simulink model "MMS_ESC_K_B_SM"  (R2019b)
settings: Solver=ode4  StartTime=par.sym.TStart  StopTime=par.sym.TStop  FixedStep=par.sym.max_dt  MaxStep=par.sym.max_dt  RelTol=1e-3
undefined symbols (not defined in the file): b, B_0, beta_B, beta_K, k, K_0, k_B, k_K, m, N_delay, par, rho_B, rho_K, T_tran, W_K, w_wav
libraries: simulink x2
settings Model: Creator=Vitù  LastModifiedBy=User
settings DataIOCC: SaveFormat=Array  SaveOutput=off  SignalLogging=off  DSMLogging=off  ReturnWorkspaceOutputs=off  TimeSaveName=TIME  OutputSaveName=Yout  OutputOption=SpecifiedOutputTimes  OutputTimes=[par.sym.TStart:par.sym.Outputdt:par.sym.TStop]
settings OptimizationCC: ExpressionDepthLimit=2147483647  LifeSpan=inf
settings DebuggingCC: UnderspecifiedInitializationDetection=Classic  MergeDetectMultiDrivingBlocksExec=none  SolverPrmCheckMsg=warning  AllowSymbolicDim=off  StateNameClashWarn=warning  SFUnexpectedBacktrackingDiag=warning  SFNoUnconditionalDefaultTransitionDiag=warning  SFExecutionAtInitializationDiag=none  ArithmeticOperatorsInVariantConditions=warning
settings HardwareCC: ProdBitPerPointer=32  ProdBitPerSizeT=32  ProdBitPerPtrDiffT=32  ProdLargestAtomicFloat=None  ProdIntDivRoundTo=Undefined  ProdEndianess=Unspecified  ProdWordSize=32  ProdHWDeviceType=32-bit Generic
settings ModelReferenceCC: PropagateSignalLabelsOutOfModel=off
settings SFSimCC: SimUseLocalCustomCode=off  CustomCodeUndefinedFunction=UseInterfaceOnly
settings RTWCC: RTWUseLocalCustomCode=off
settings CodeAppCC: StateflowObjectComments=on
settings GRTTargetCC: TargetLangStandard=C89/C90 (ANSI)  GeneratePreprocessorConditionals=Disable all
settings ConfigComp: CovMetricSettings=dw  CovHtmlReporting=on  CovSaveCumulativeToWorkspaceVar=on  CovSaveSingleToWorkspaceVar=on  CovExternalEMLEnable=off  CovSFcnEnable=off
settings SimscapeCC: SimscapeNormalizeSystem=off
settings ConfigurationSet: Description=SimMechanics 2G

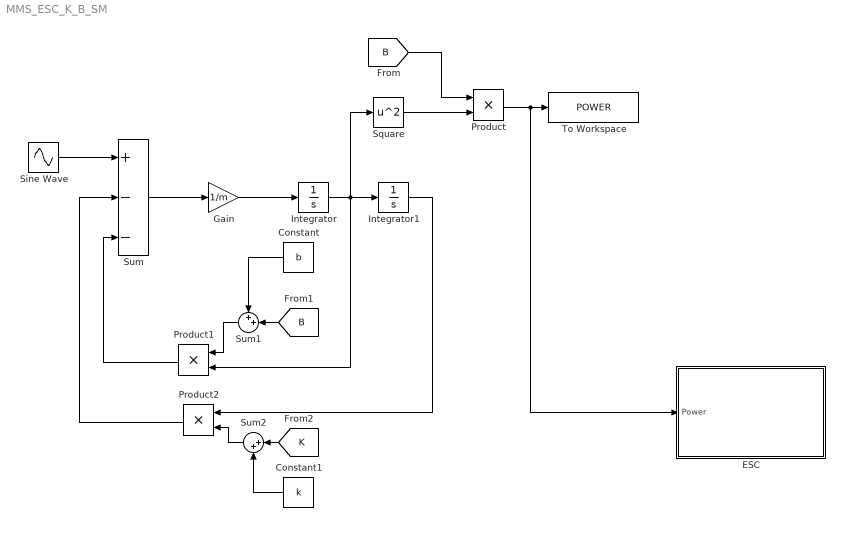
== system MMS_ESC_K_B_SM ==
  Constant : Constant  Value=b
  Constant1 : Constant  Value=k
  ESC : Subsystem
  Gain : Gain  Gain=1/m
  Integrator : Integrator
  Integrator1 : Integrator
  Product : Product
  Product1 : Product
  Product2 : Product
  Sine Wave : Sin  Amplitude=par.H  Frequency=w_wav  SampleTime=0
  Square : Math  Operator=square  SignedPower=off  SaturateOnIntegerOverflow=on
  Sum : Sum  Inputs=+--
  Sum1 : Sum  Inputs=++|
  Sum2 : Sum  Inputs=|++
  To Workspace : ToWorkspace  VariableName=POWER  SampleTime=-1
  wires:
  Integrator1/1 -> Product2/1
  Product/1 -> ESC/1(Power), To Workspace/1
  Product1/1 -> Sum/3
  Gain/1 -> Integrator/1
  Square/1 -> Product/2
  Sum/1 -> Gain/1
  Integrator/1 -> Product1/2, Square/1, Integrator1/1
  Product2/1 -> Sum/2
  Sine Wave/1 -> Sum/1
  [B] -> Product/1
  [B] -> Sum1/2
  Sum1/1 -> Product1/1
  Constant/1 -> Sum1/1
  [K] -> Sum2/1
  Sum2/1 -> Product2/2
  Constant1/1 -> Sum2/2

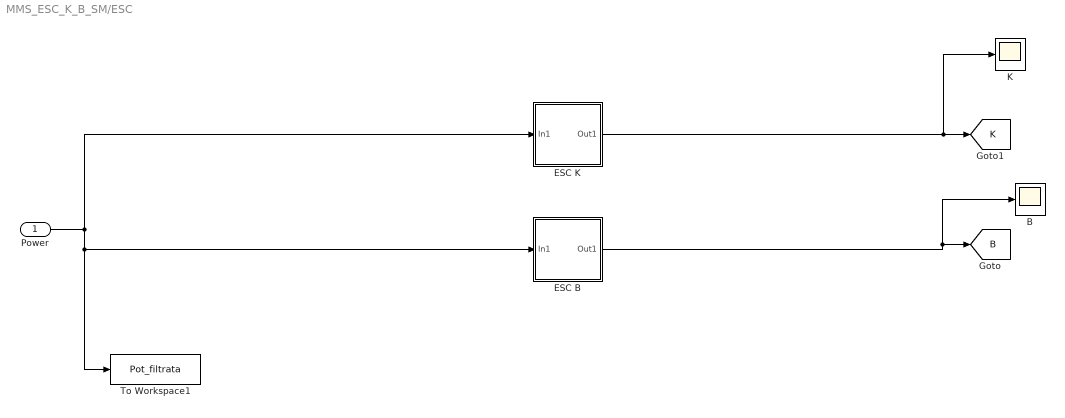
== system MMS_ESC_K_B_SM/ESC ==
  Power : Inport
  B : Scope
  ESC B : Subsystem
  ESC K : Subsystem
  K : Scope
  To Workspace1 : ToWorkspace  VariableName=Pot_filtrata  SampleTime=-1
  tag scope: B=global, K=global
  wires:
  ESC B/1(Out1) -> B/1, [B]
  ESC K/1(Out1) -> K/1, [K]
  Power/1 -> To Workspace1/1, ESC B/1(In1), ESC K/1(In1)

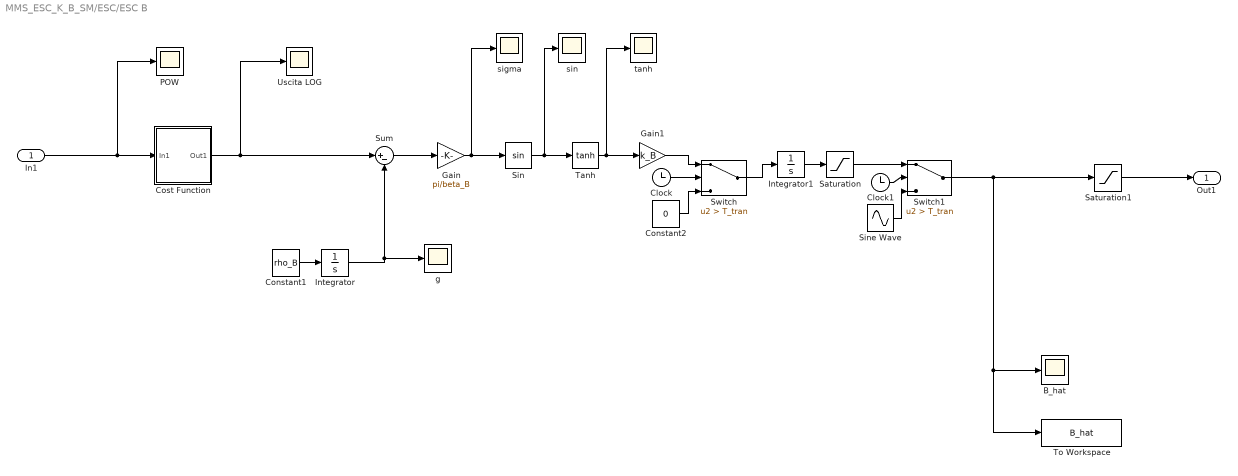
== system MMS_ESC_K_B_SM/ESC/ESC B ==
  In1 : Inport
  B_hat : Scope
  Clock : Clock
  Clock1 : Clock
  Constant1 : Constant  Value=rho_B
  Constant2 : Constant  Value=0
  Cost Function : Subsystem
  Gain : Gain  Gain=pi/beta_B
  Gain1 : Gain  Gain=k_B
  Integrator : Integrator
  Integrator1 : Integrator  InitialCondition=B_0
  POW : Scope
  Saturation : Saturate  UpperLimit=inf  LowerLimit=5
  Saturation1 : Saturate  UpperLimit=inf  LowerLimit=-b
  Sin : Trigonometry
  Sine Wave : Sin  Amplitude=5  Bias=B_0  Frequency=w_wav  SampleTime=0
  Sum : Sum  Inputs=|+-
  Switch : Switch  Criteria=u2 > Threshold  Threshold=T_tran
  Switch1 : Switch  Criteria=u2 > Threshold  Threshold=T_tran
  Tanh : Trigonometry  Operator=tanh
  To Workspace : ToWorkspace  VariableName=B_hat  SampleTime=-1
  Uscita LOG : Scope
  g : Scope
  sigma : Scope
  sin : Scope
  tanh : Scope
  Out1 : Outport
  wires:
  Integrator/1 -> g/1, Sum/2
  Gain/1 -> sigma/1, Sin/1
  Switch1/1 -> Saturation1/1, To Workspace/1, B_hat/1
  Sin/1 -> sin/1, Tanh/1
  Tanh/1 -> tanh/1, Gain1/1
  Switch/1 -> Integrator1/1
  Cost Function/1(Out1) -> Uscita LOG/1, Sum/1
  Sine Wave/1 -> Switch1/3
  Clock1/1 -> Switch1/2
  Constant1/1 -> Integrator/1
  Gain1/1 -> Switch/1
  Sum/1 -> Gain/1
  Clock/1 -> Switch/2
  Constant2/1 -> Switch/3
  Integrator1/1 -> Saturation/1
  In1/1 -> POW/1, Cost Function/1(In1)
  Saturation/1 -> Switch1/1
  Saturation1/1 -> Out1/1

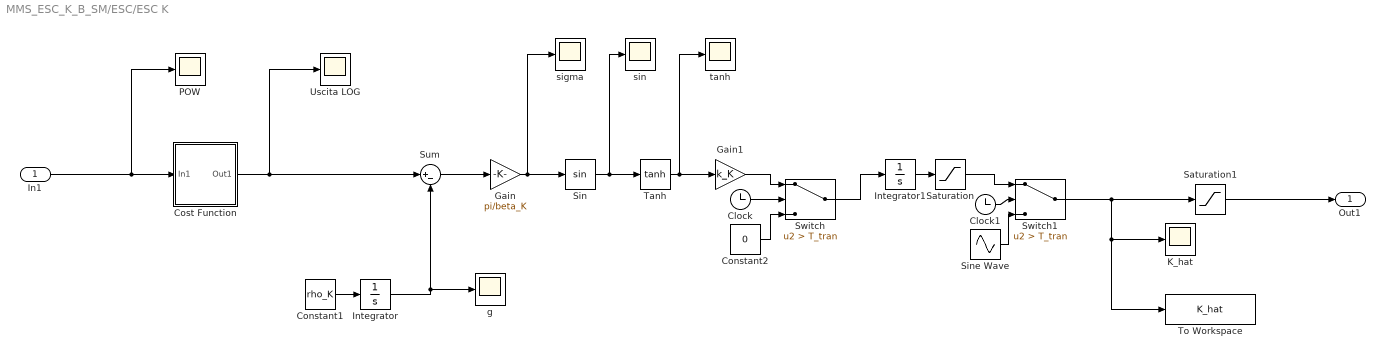
== system MMS_ESC_K_B_SM/ESC/ESC K ==
  In1 : Inport
  Clock : Clock
  Clock1 : Clock
  Constant1 : Constant  Value=rho_K
  Constant2 : Constant  Value=0
  Cost Function : Subsystem
  Gain : Gain  Gain=pi/beta_K
  Gain1 : Gain  Gain=k_K
  Integrator : Integrator
  Integrator1 : Integrator  InitialCondition=K_0
  K_hat : Scope
  POW : Scope
  Saturation : Saturate  UpperLimit=inf  LowerLimit=100
  Saturation1 : Saturate  UpperLimit=inf  LowerLimit=-k
  Sin : Trigonometry
  Sine Wave : Sin  Amplitude=50  Bias=K_0  Frequency=w_wav  SampleTime=0
  Sum : Sum  Inputs=|+-
  Switch : Switch  Criteria=u2 > Threshold  Threshold=T_tran
  Switch1 : Switch  Criteria=u2 > Threshold  Threshold=T_tran
  Tanh : Trigonometry  Operator=tanh
  To Workspace : ToWorkspace  VariableName=K_hat  SampleTime=-1
  Uscita LOG : Scope
  g : Scope
  sigma : Scope
  sin : Scope
  tanh : Scope
  Out1 : Outport
  wires:
  Integrator/1 -> g/1, Sum/2
  Gain/1 -> sigma/1, Sin/1
  Switch1/1 -> Saturation1/1, To Workspace/1, K_hat/1
  Sin/1 -> sin/1, Tanh/1
  Tanh/1 -> tanh/1, Gain1/1
  Switch/1 -> Integrator1/1
  Cost Function/1(Out1) -> Uscita LOG/1, Sum/1
  Sine Wave/1 -> Switch1/3
  Clock1/1 -> Switch1/2
  Constant1/1 -> Integrator/1
  Gain1/1 -> Switch/1
  Sum/1 -> Gain/1
  Clock/1 -> Switch/2
  Constant2/1 -> Switch/3
  Integrator1/1 -> Saturation/1
  In1/1 -> POW/1, Cost Function/1(In1)
  Saturation/1 -> Switch1/1
  Saturation1/1 -> Out1/1

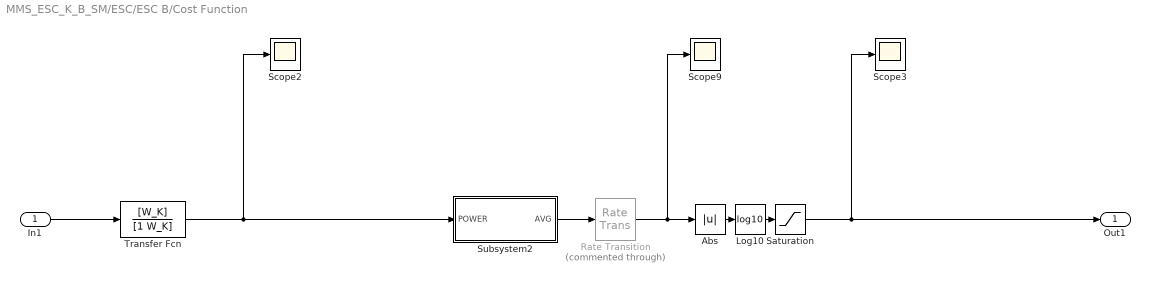
== system MMS_ESC_K_B_SM/ESC/ESC B/Cost Function ==
  In1 : Inport
  Abs : Abs
  Log10 : Math  Operator=log10  SignedPower=off  SaturateOnIntegerOverflow=on
  Rate Transition : RateTransition  Commented=through
  Saturation : Saturate  UpperLimit=inf  LowerLimit=-40
  Scope2 : Scope
  Scope3 : Scope
  Scope9 : Scope
  Subsystem2 : Subsystem
  Transfer Fcn : TransferFcn  Numerator=[W_K]  Denominator=[1 W_K]
  Out1 : Outport
  wires:
  Subsystem2/1(AVG) -> Rate Transition/1
  Rate Transition/1 -> Abs/1, Scope9/1
  In1/1 -> Transfer Fcn/1
  Transfer Fcn/1 -> Subsystem2/1(POWER), Scope2/1
  Abs/1 -> Log10/1
  Log10/1 -> Saturation/1
  Saturation/1 -> Out1/1, Scope3/1

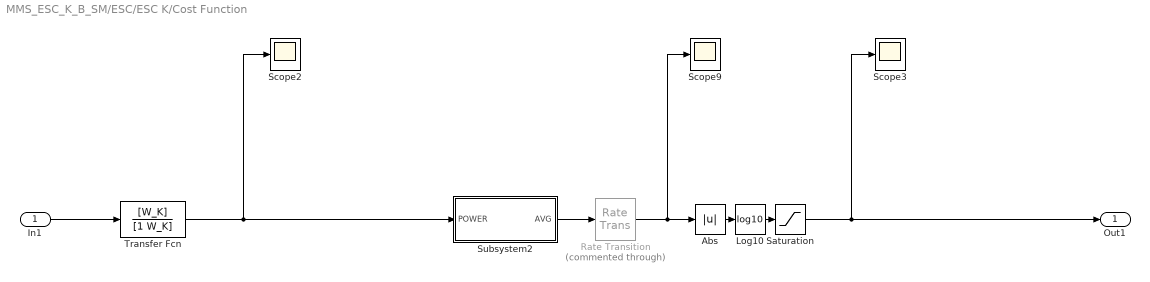
== system MMS_ESC_K_B_SM/ESC/ESC K/Cost Function ==
  In1 : Inport
  Abs : Abs
  Log10 : Math  Operator=log10  SignedPower=off  SaturateOnIntegerOverflow=on
  Rate Transition : RateTransition  Commented=through
  Saturation : Saturate  UpperLimit=inf  LowerLimit=-40
  Scope2 : Scope
  Scope3 : Scope
  Scope9 : Scope
  Subsystem2 : Subsystem
  Transfer Fcn : TransferFcn  Numerator=[W_K]  Denominator=[1 W_K]
  Out1 : Outport
  wires:
  Subsystem2/1(AVG) -> Rate Transition/1
  Rate Transition/1 -> Abs/1, Scope9/1
  In1/1 -> Transfer Fcn/1
  Transfer Fcn/1 -> Subsystem2/1(POWER), Scope2/1
  Abs/1 -> Log10/1
  Log10/1 -> Saturation/1
  Saturation/1 -> Out1/1, Scope3/1

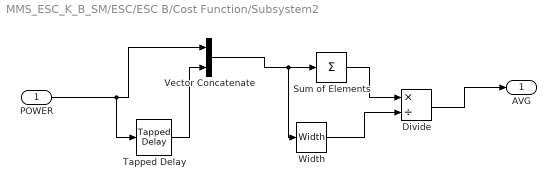
== system MMS_ESC_K_B_SM/ESC/ESC B/Cost Function/Subsystem2 ==
  POWER : Inport
  Divide : Product  Inputs=*/
  Sum of Elements : Sum  Inputs=+
  Tapped Delay : simulink/Discrete/Tapped Delay  vinit=0  samptime=-1  NumDelays=N_delay  DelayOrder=Oldest  includeCurrent=off
  Vector Concatenate : Concatenate
  Width : Width
  AVG : Outport
  wires:
  POWER/1 -> Tapped Delay/1, Vector Concatenate/1
  Tapped Delay/1 -> Vector Concatenate/2
  Vector Concatenate/1 -> Width/1, Sum of Elements/1
  Sum of Elements/1 -> Divide/1
  Width/1 -> Divide/2
  Divide/1 -> AVG/1

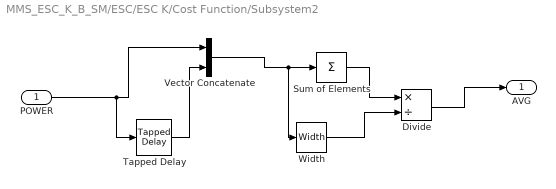
== system MMS_ESC_K_B_SM/ESC/ESC K/Cost Function/Subsystem2 ==
  POWER : Inport
  Divide : Product  Inputs=*/
  Sum of Elements : Sum  Inputs=+
  Tapped Delay : simulink/Discrete/Tapped Delay  vinit=0  samptime=-1  NumDelays=N_delay  DelayOrder=Oldest  includeCurrent=off
  Vector Concatenate : Concatenate
  Width : Width
  AVG : Outport
  wires:
  POWER/1 -> Tapped Delay/1, Vector Concatenate/1
  Tapped Delay/1 -> Vector Concatenate/2
  Vector Concatenate/1 -> Width/1, Sum of Elements/1
  Sum of Elements/1 -> Divide/1
  Width/1 -> Divide/2
  Divide/1 -> AVG/1
